simulink model "Zadatak1_Provjera"  (R2018a)
settings: Solver=ode45  StartTime=0.0  StopTime=10.0  RelTol=1e-3
undefined symbols (not defined in the file or in its folder): j
libraries: powerlib x28
settings Model: Creator=Panjevic  LastModifiedBy=Panjevic

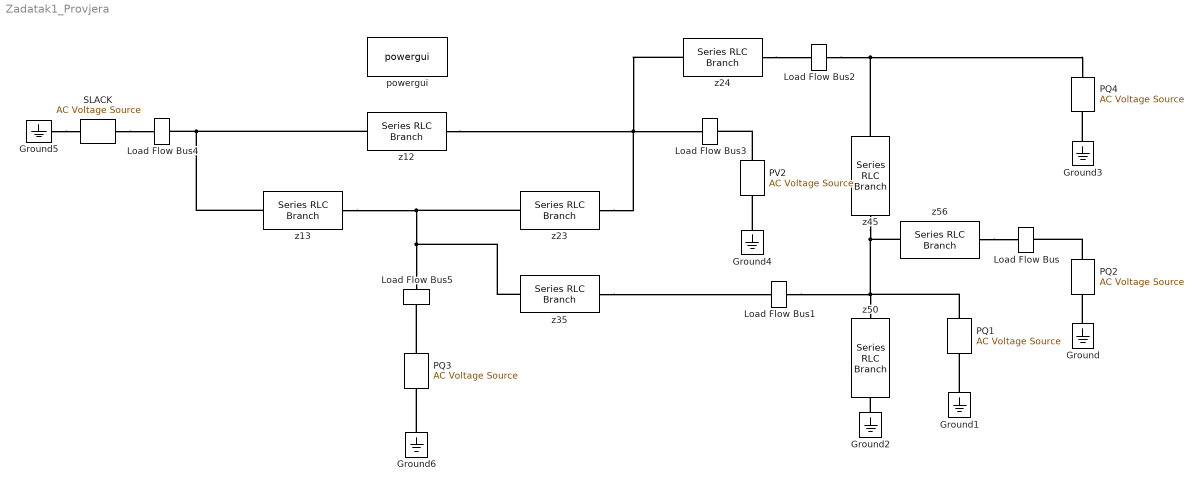
== system Zadatak1_Provjera ==
  Ground{,1..6} (7 alike) : powerlib/Elements/Ground  LConnTagsString=a
  Load Flow Bus : powerlib/Measurements/Load Flow Bus  LConnTagsString=a  RConnTagsString=a  Phases=A  Connectors=on both sides  ID=BUS_6  Vbase=1  Vref=1  Vangle=0  VLF=0.5364  VLFb=NaN  VLFc=NaN  angleLF=69.09  angleLFb=NaN  angleLFc=NaN
      settings: SourceProductName=Simscape Power Systems
  Load Flow Bus1 : powerlib/Measurements/Load Flow Bus  LConnTagsString=a  RConnTagsString=a  Phases=A  Connectors=on both sides  ID=BUS_5  Vbase=1  Vref=1  Vangle=0  VLF=0.6959  VLFb=NaN  VLFc=NaN  angleLF=66.41  angleLFb=NaN  angleLFc=NaN
      settings: SourceProductName=Simscape Power Systems
  Load Flow Bus2 : powerlib/Measurements/Load Flow Bus  LConnTagsString=a  RConnTagsString=a  Phases=A  Connectors=on both sides  ID=BUS_4  Vbase=1  Vref=1  Vangle=0  VLF=0.9818  VLFb=NaN  VLFc=NaN  angleLF=66.2  angleLFb=NaN  angleLFc=NaN
      settings: SourceProductName=Simscape Power Systems
  Load Flow Bus3 : powerlib/Measurements/Load Flow Bus  LConnTagsString=a  RConnTagsString=a  Phases=A  Connectors=on both sides  ID=BUS_2  Vbase=1  Vref=1.02  Vangle=0  VLF=1.02  VLFb=NaN  VLFc=NaN  angleLF=61.59  angleLFb=NaN  angleLFc=NaN
      settings: SourceProductName=Simscape Power Systems
  Load Flow Bus4 : powerlib/Measurements/Load Flow Bus  LConnTagsString=a  RConnTagsString=a  Phases=A  Connectors=on both sides  ID=BUS_1  Vbase=1  Vref=abs(1/sqrt(3)+j*sqrt(2/3))  Vangle=angle(1/sqrt(3)+j*sqrt(2/3))*180/pi  VLF=1  VLFb=NaN  VLFc=NaN  angleLF=54.74  angleLFb=NaN  angleLFc=NaN
      settings: SourceProductName=Simscape Power Systems
  Load Flow Bus5 : powerlib/Measurements/Load Flow Bus  LConnTagsString=a  RConnTagsString=a  Phases=A  Connectors=on both sides  ID=BUS_3  Vbase=1  Vref=0.9  Vangle=0  VLF=1.026  VLFb=NaN  VLFc=NaN  angleLF=58.96  angleLFb=NaN  angleLFc=NaN
      settings: SourceProductName=Simscape Power Systems
  PQ1 : powerlib/Electrical Sources/AC Voltage Source  Amplitude=0.695888*1*sqrt(2)  Phase=66.4101  Frequency=50  SampleTime=0  Measurements=Voltage  BusType=PQ  Pref=0  Qref=0  Qmin=-inf  Qmax=+inf
  PQ2 : powerlib/Electrical Sources/AC Voltage Source  Amplitude=0.5364*1*sqrt(2)  Phase=69.0934  Frequency=50  SampleTime=0  Measurements=Voltage  BusType=PQ  Pref=1.3  Qref=0.3  Qmin=-inf  Qmax=+inf
  PQ3 : powerlib/Electrical Sources/AC Voltage Source  Amplitude=1.02562*1*sqrt(2)  Phase=58.9615  Frequency=50  SampleTime=0  Measurements=Voltage  BusType=PQ  Pref=-1.4  Qref=-0.9  Qmin=-inf  Qmax=+inf
  PQ4 : powerlib/Electrical Sources/AC Voltage Source  Amplitude=0.981754*1*sqrt(2)  Phase=66.2019  Frequency=50  SampleTime=0  Measurements=Voltage  BusType=PQ  Pref=-2  Qref=0  Qmin=-inf  Qmax=+inf
  PV2 : powerlib/Electrical Sources/AC Voltage Source  Amplitude=1.02*1*sqrt(2)  Phase=61.5899  Frequency=50  SampleTime=0  Measurements=Voltage  BusType=PV  Pref=3  Qref=-0.9  Qmin=-inf  Qmax=+inf
  SLACK : powerlib/Electrical Sources/AC Voltage Source  Amplitude=1*1*sqrt(2)  Phase=54.7356  Frequency=50  SampleTime=0  Measurements=None  BusType=swing  Pref=-1.4  Qref=-0.9  Qmin=-inf  Qmax=+inf
  powergui : powerlib/powergui  Priority=1  SimulationMode=Phasor  SampleTime=50e-6  frequency=50  Iterations=50  frequencyindice=50  Pbase=100e6  ErrMax=0.0001  UnitsV=kV  UnitsW=MW  buscounter=0  FunctionMessages=off  echomessages=off  EnableUseOfTLC=off  CurrentSourceSwitches=off  DisableSnubberDevices=off  DisableRonSwitches=off  DisableVfSwitches=off  DisplayEquations=off  SolverType=Tustin/Backward Euler (TBE)  Interpol=off  ExternalGateDelay=off  methode=off  Ts=100  x0status=blocks  SPID=on  SwTol=0  HookPort=off  RestoreLinks=warning  ResistiveCurrentMeasurement=off  Frange=[0:2:500]  Ylog=off  Xlog=on  ShowGrid=off  save=off  variable=ZData  structure=0  ZoomFFT=off  StartTime=0.0  cycles=1  DisplayStyle=1  fundamental=60  FreqAxis=off  MaxFrequency=1000  frequencyindicesteady=1  RmsSteady=1  display=off
  "z12 " : powerlib/Elements/Series RLC Branch  LConnTagsString=__new0  RConnTagsString=__new0  BranchType=RL  Resistance=0.05  Inductance=0.1/(2*pi*50)  SetiL0=off  InitialCurrent=0  Capacitance=0.1  Setx0=off  InitialVoltage=0  Measurements=None
  z13 : powerlib/Elements/Series RLC Branch  LConnTagsString=__new0  RConnTagsString=__new0  BranchType=RL  Resistance=0.025  Inductance=0.03/(2*pi*50)  SetiL0=off  InitialCurrent=0  Capacitance=0.1  Setx0=off  InitialVoltage=0  Measurements=None
  z23 : powerlib/Elements/Series RLC Branch  LConnTagsString=__new0  RConnTagsString=__new0  BranchType=RL  Resistance=0.02  Inductance=0.02/(2*pi*50)  SetiL0=off  InitialCurrent=0  Capacitance=0.1  Setx0=off  InitialVoltage=0  Measurements=None
  z24 : powerlib/Elements/Series RLC Branch  LConnTagsString=__new0  RConnTagsString=__new0  BranchType=RC  Resistance=0.06  Inductance=1e-3  SetiL0=off  InitialCurrent=0  Capacitance=1/(0.1*2*pi*50)  Setx0=off  InitialVoltage=0  Measurements=None
  "z35 " : powerlib/Elements/Series RLC Branch  LConnTagsString=__new0  RConnTagsString=__new0  BranchType=RL  Resistance=0.54  Inductance=0.1/(2*pi*50)  SetiL0=off  InitialCurrent=0  Capacitance=0.1  Setx0=off  InitialVoltage=0  Measurements=None
  z45 : powerlib/Elements/Series RLC Branch  LConnTagsString=__new0  RConnTagsString=__new0  BranchType=R  Resistance=0.1  Inductance=1e-3  SetiL0=off  InitialCurrent=0  Capacitance=1e-6  Setx0=off  InitialVoltage=0  Measurements=None
  z50 : powerlib/Elements/Series RLC Branch  LConnTagsString=__new0  RConnTagsString=__new0  BranchType=R  Resistance=0.5  Inductance=1e-3  SetiL0=off  InitialCurrent=0  Capacitance=1e-6  Setx0=off  InitialVoltage=0  Measurements=None
  z56 : powerlib/Elements/Series RLC Branch  LConnTagsString=__new0  RConnTagsString=__new0  BranchType=R  Resistance=0.08  Inductance=1e-3  SetiL0=off  InitialCurrent=0  Capacitance=1e-6  Setx0=off  InitialVoltage=0  Measurements=None
  connections:
  Ground/LConn1 -- PQ2/LConn1
  Ground1/LConn1 -- PQ1/LConn1
  PQ1/RConn1 -- z45/LConn1 -- z56/RConn1 -- Load Flow Bus1/RConn1 -- z50/LConn1
  Ground2/LConn1 -- z50/RConn1
  PQ2/RConn1 -- Load Flow Bus/RConn1
  z56/LConn1 -- Load Flow Bus/LConn1
  Ground3/LConn1 -- PQ4/LConn1
  Load Flow Bus2/RConn1 -- z45/RConn1 -- PQ4/RConn1
  z24/RConn1 -- Load Flow Bus2/LConn1
  Ground4/LConn1 -- PV2/LConn1
  PV2/RConn1 -- Load Flow Bus3/RConn1
  z24/LConn1 -- z23/RConn1 -- Load Flow Bus3/LConn1 -- "z12 "/RConn1
  Ground5/LConn1 -- SLACK/LConn1
  SLACK/RConn1 -- Load Flow Bus4/LConn1
  "z12 "/LConn1 -- z13/LConn1 -- Load Flow Bus4/RConn1
  z13/RConn1 -- z23/LConn1 -- "z35 "/LConn1 -- Load Flow Bus5/LConn1
  Ground6/LConn1 -- PQ3/LConn1
  PQ3/RConn1 -- Load Flow Bus5/RConn1
  "z35 "/RConn1 -- Load Flow Bus1/LConn1
